simulink model "Evaluation"  (Simulink 7.6)
settings: Solver=ode45  StartTime=0.0  StopTime=10.0  RelTol=1e-3
libraries: powerlib_extras x1, simulink x1
settings Model: Creator=Zsolt  LastModifiedBy=Zsolt
settings HardwareCC: TargetIntDivRoundTo=Zero  TargetEndianess=LittleEndian  TargetHWDeviceType=MATLAB Host  ProdEqTarget=off
settings RTWCC: SystemTargetFile=rsim.tlc  TemplateMakefile=rsim_default_tmf  Description=Rapid Simulation Target  ProcessScript=rsim_make_rtw_hook
settings RSimTargetCC: TargetFunctionLibrary=ANSI_C  ERTMultiwordTypeDef=System defined  ERTCodeCoverageTool=None  ERTMultiwordLength=256  IsPILTarget=off  EnableShiftOperators=on  PortableWordSizes=off

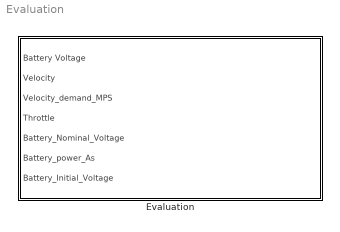
== system Evaluation ==
  Evaluation : Subsystem

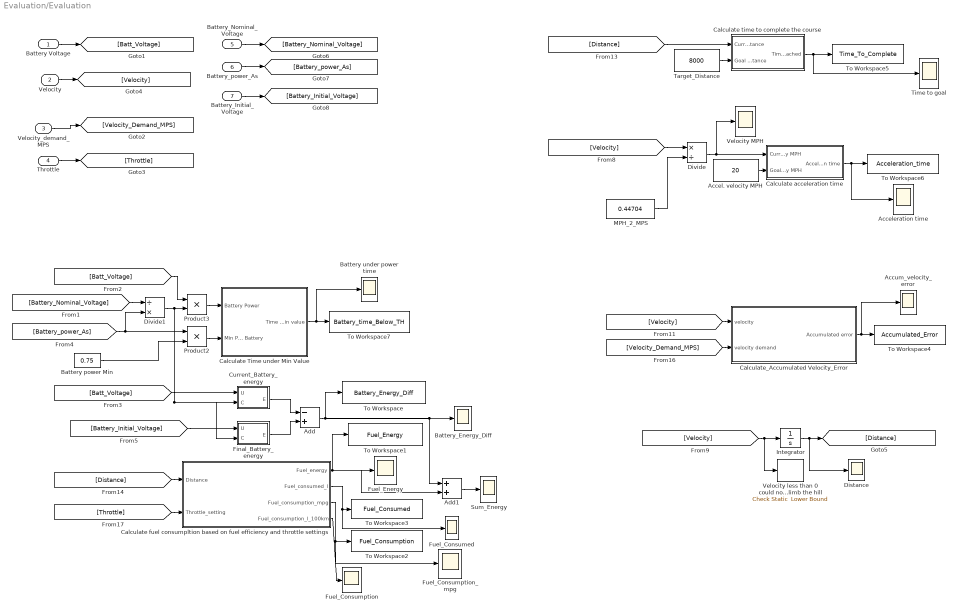
== system Evaluation/Evaluation ==
  Battery Voltage : Inport
  Velocity : Inport  Port=2
  Velocity_demand_MPS : Inport  Port=3
  Throttle : Inport  Port=4
  Battery_Nominal_Voltage : Inport  Port=5
  Battery_power_As : Inport  Port=6
  Battery_Initial_Voltage : Inport  Port=7
  Accel. velocity MPH : Constant  Value=20
  Acceleration time : Scope
      settings: TimeRange=500  YMin=0  YMax=10  SaveName=ScopeData15
  Accum_velocity_error : Scope
      settings: TimeRange=500  YMin=0  YMax=500  SaveName=ScopeData6
  Add : Sum  Inputs=-+
  Add1 : Sum
  Battery power Min : Constant  Value=0.75
  Battery under power time : Scope
      settings: TimeRange=500  YMin=0  YMax=400
  Battery_Energy_Diff : Scope
      settings: TimeRange=500  YMin=-500000  YMax=2000000  SaveName=ScopeData20
  Calculate Time under Min Value : Subsystem
  Calculate acceleration time : Subsystem
  Calculate time to complete the course : Subsystem
  Calculate fuel consumpltion based on fuel efficiency and throttle settings : Subsystem
  Calculate_Accumulated Velocity_Error : Subsystem
  Current_Battery_energy : Subsystem
  Distance : Scope
      settings: TimeRange=500  YMin=0  YMax=12000  SaveName=ScopeData8
  Divide : Product  Inputs=*/
  Divide1 : Product  Inputs=/*
  Final_Battery_energy : Subsystem
  Fuel_Consumed : Scope
      settings: TimeRange=500  YMin=0  YMax=20  SaveName=ScopeData21
  Fuel_Consumption : Scope
      settings: TimeRange=500  YMin=0  YMax=4000  SaveName=ScopeData22
  Fuel_Consumption_mpg : Scope
      settings: TimeRange=500  YMin=0  YMax=2  SaveName=ScopeData23
  Fuel_Energy : Scope
      settings: TimeRange=500  YMin=0  YMax=300000000  SaveName=ScopeData24
  Integrator : Integrator
  MPH_2_MPS : Constant  Value=0.44704
  Product2 : Product  RndMeth=Zero
  Product3 : Product  RndMeth=Zero
  Sum_Energy : Scope
      settings: TimeRange=500  YMin=0  YMax=14000  SaveName=ScopeData25
  Target_Distance : Constant  Value=8000
  Time to goal : Scope
      settings: TimeRange=500  YMin=0  YMax=500  SaveName=ScopeData5
  To Workspace : ToWorkspace  VariableName=Battery_Energy_Diff  SampleTime=-1  SaveFormat=Structure
  To Workspace1 : ToWorkspace  VariableName=Fuel_Energy  SampleTime=-1  SaveFormat=Structure
  To Workspace2 : ToWorkspace  VariableName=Fuel_Consumption  SampleTime=-1  SaveFormat=Structure
  To Workspace3 : ToWorkspace  VariableName=Fuel_Consumed  SampleTime=-1  SaveFormat=Structure
  To Workspace4 : ToWorkspace  VariableName=Accumulated_Error  SampleTime=-1  SaveFormat=Structure
  To Workspace5 : ToWorkspace  VariableName=Time_To_Complete  SampleTime=-1  SaveFormat=Structure
  To Workspace6 : ToWorkspace  VariableName=Acceleration_time  SampleTime=-1  SaveFormat=Structure
  To Workspace7 : ToWorkspace  VariableName=Battery_time_Below_TH  SampleTime=-1  SaveFormat=Structure
  Velocity MPH : Scope
      settings: TimeRange=500  YMin=0  YMax=60  SaveName=ScopeData13
  Velocity less than 0 could not climb the hill : simulink/Model Verification/Check Static  Lower Bound  Description=0 <= u  SystemSampleTime=-1  min=0  min_included=on  enabled=on  stopWhenAssertionFail=on  export=off  icon=graphic
  wires:
  MPH_2_MPS/1 -> Divide/2
  [Velocity] -> Divide/1
  Divide/1 -> Calculate acceleration time/1(Current Velocity MPH), Velocity MPH/1
  Calculate acceleration time/1(Acceleration time) -> Acceleration time/1, To Workspace6/1
  Accel. velocity MPH/1 -> Calculate acceleration time/2(Goal Velocity MPH)
  Product3/1 -> Calculate Time under Min Value/1(Battery Power)
  Battery power Min/1 -> Product2/2
  [Battery_power_As] -> Product2/1, Divide1/2
  Product2/1 -> Calculate Time under Min Value/2(Min Power in Battery)
  Calculate Time under Min Value/1(Time under Min value) -> Battery under power time/1, To Workspace7/1
  Calculate fuel consumpltion based on fuel efficiency and throttle settings/3(Fuel_consumption_mpg) -> Fuel_Consumption_mpg/1, To Workspace2/1
  Calculate fuel consumpltion based on fuel efficiency and throttle settings/2(Fuel_consumed_l) -> Fuel_Consumed/1, To Workspace3/1
  Calculate fuel consumpltion based on fuel efficiency and throttle settings/1(Fuel_energy) -> Fuel_Energy/1, To Workspace1/1, Add1/2
  Calculate fuel consumpltion based on fuel efficiency and throttle settings/4(Fuel_consumption_l_100km) -> Fuel_Consumption/1
  Add1/1 -> Sum_Energy/1
  Add/1 -> Battery_Energy_Diff/1, To Workspace/1, Add1/1
  Final_Battery_energy/1(E) -> Add/2
  Current_Battery_energy/1(E) -> Add/1
  [Battery_Initial_Voltage] -> Final_Battery_energy/1(U)
  [Batt_Voltage] -> Current_Battery_energy/1(U)
  [Distance] -> Calculate fuel consumpltion based on fuel efficiency and throttle settings/1(Distance)
  [Batt_Voltage] -> Product3/1
  Divide1/1 -> Product3/2, Final_Battery_energy/2(C), Current_Battery_energy/2(C)
  [Battery_Nominal_Voltage] -> Divide1/1
  [Throttle] -> Calculate fuel consumpltion based on fuel efficiency and throttle settings/2(Throttle_setting)
  Calculate time to complete the course/1(Time when reached) -> Time to goal/1, To Workspace5/1
  Target_Distance/1 -> Calculate time to complete the course/2(Goal Distance)
  [Distance] -> Calculate time to complete the course/1(Current Distance)
  Calculate_Accumulated Velocity_Error/1(Accumulated error) -> Accum_velocity_error/1, To Workspace4/1
  [Velocity] -> Calculate_Accumulated Velocity_Error/1(velocity)
  [Velocity_Demand_MPS] -> Calculate_Accumulated Velocity_Error/2(velocity demand)
  [Velocity] -> Integrator/1, Velocity less than 0 could not climb the hill/1
  Integrator/1 -> [Distance], Distance/1
  Battery Voltage/1 -> [Batt_Voltage]
  Velocity/1 -> [Velocity]
  Velocity_demand_MPS/1 -> [Velocity_Demand_MPS]
  Throttle/1 -> [Throttle]
  Battery_Nominal_Voltage/1 -> [Battery_Nominal_Voltage]
  Battery_power_As/1 -> [Battery_power_As]
  Battery_Initial_Voltage/1 -> [Battery_Initial_Voltage]

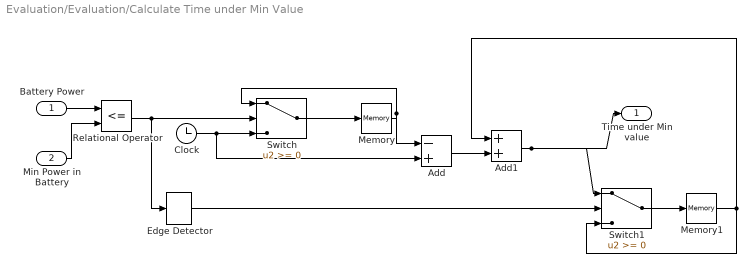
== system Evaluation/Evaluation/Calculate Time under Min Value ==
  Battery Power : Inport
  Min Power in Battery : Inport  Port=2
  Add : Sum  Inputs=-+
  Add1 : Sum
  Clock : Clock
      settings: Decimation=10
  Edge Detector : powerlib_extras/Control  Blocks/Edge Detector  DialogController=POWERSYS.PowerSysDialog  SystemSampleTime=-1  model=Falling  ic=0
  Memory : Memory
  Memory1 : Memory
  Relational Operator : RelationalOperator  Operator=<=  OutDataTypeStr=boolean
  Switch : Switch
  Switch1 : Switch
  Time under Min value : Outport
  wires:
  Switch/1 -> Memory/1
  Memory/1 -> Switch/1, Add/1
  Relational Operator/1 -> Switch/2, Edge Detector/1
  Clock/1 -> Switch/3, Add/2
  Add/1 -> Add1/2
  Switch1/1 -> Memory1/1
  Edge Detector/1 -> Switch1/2
  Memory1/1 -> Switch1/3, Add1/1
  Add1/1 -> Switch1/1, Time under Min value/1
  Battery Power/1 -> Relational Operator/1
  Min Power in Battery/1 -> Relational Operator/2

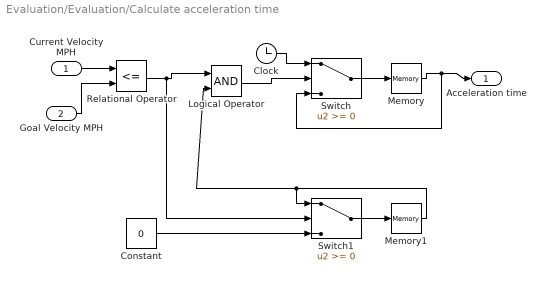
== system Evaluation/Evaluation/Calculate acceleration time ==
  Current Velocity MPH : Inport
  Goal Velocity MPH : Inport  Port=2
  Clock : Clock
      settings: Decimation=10
  Constant : Constant  Value=0
  Logical Operator : Logic  AllPortsSameDT=off  OutDataTypeStr=boolean
  Memory : Memory
  Memory1 : Memory  X0=1
  Relational Operator : RelationalOperator  Operator=<=  OutDataTypeStr=boolean
  Switch : Switch
  Switch1 : Switch
  Acceleration time : Outport
  wires:
  Goal Velocity MPH/1 -> Relational Operator/2
  Current Velocity MPH/1 -> Relational Operator/1
  Memory/1 -> Acceleration time/1, Switch/3
  Switch/1 -> Memory/1
  Memory1/1 -> Switch1/1, Logical Operator/2
  Switch1/1 -> Memory1/1
  Relational Operator/1 -> Logical Operator/1, Switch1/2
  Logical Operator/1 -> Switch/2
  Constant/1 -> Switch1/3
  Clock/1 -> Switch/1

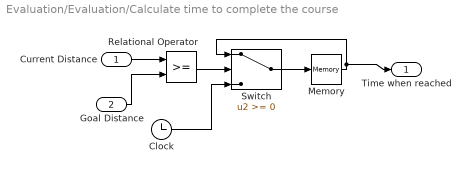
== system Evaluation/Evaluation/Calculate time to complete the course ==
  Current Distance : Inport
  Goal Distance : Inport  Port=2
  Clock : Clock
      settings: Decimation=10
  Memory : Memory
  Relational Operator : RelationalOperator  OutDataTypeStr=boolean
  Switch : Switch
  Time when reached : Outport
  wires:
  Switch/1 -> Memory/1
  Memory/1 -> Switch/1, Time when reached/1
  Relational Operator/1 -> Switch/2
  Clock/1 -> Switch/3
  Current Distance/1 -> Relational Operator/1
  Goal Distance/1 -> Relational Operator/2

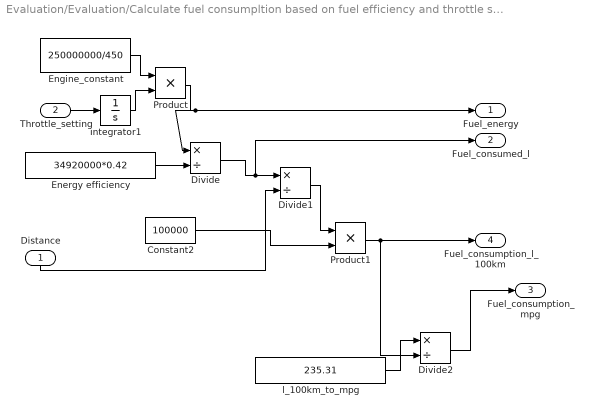
== system Evaluation/Evaluation/Calculate fuel consumpltion based on fuel efficiency and throttle settings ==
  Distance : Inport
  Throttle_setting : Inport  Port=2
  Constant2 : Constant  Value=100000
  Divide : Product  Inputs=*/
  Divide1 : Product  Inputs=*/
  Divide2 : Product  Inputs=*/
  Energy efficiency : Constant  Value=34920000*0.42
  Engine_constant : Constant  Value=250000000/450
  Integrator1 : Integrator
  Product : Product  RndMeth=Zero
  Product1 : Product  RndMeth=Zero
  l_100km_to_mpg : Constant  Value=235.31
  Fuel_energy : Outport
  Fuel_consumed_l : Outport  Port=2
  Fuel_consumption_mpg : Outport  Port=3
  Fuel_consumption_l_100km : Outport  Port=4
  wires:
  Integrator1/1 -> Product/2
  Product/1 -> Divide/1, Fuel_energy/1
  Engine_constant/1 -> Product/1
  Energy efficiency/1 -> Divide/2
  Divide/1 -> Divide1/1, Fuel_consumed_l/1
  Divide1/1 -> Product1/1
  Constant2/1 -> Product1/2
  Throttle_setting/1 -> Integrator1/1
  Distance/1 -> Divide1/2
  Product1/1 -> Fuel_consumption_l_100km/1, Divide2/2
  Divide2/1 -> Fuel_consumption_mpg/1
  l_100km_to_mpg/1 -> Divide2/1

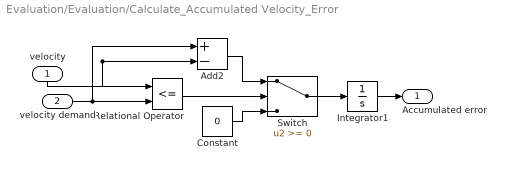
== system Evaluation/Evaluation/Calculate_Accumulated Velocity_Error ==
  velocity : Inport
  velocity demand : Inport  Port=2
  Add2 : Sum  Inputs=+-
  Constant : Constant  Value=0
  Integrator1 : Integrator
  Relational Operator : RelationalOperator  Operator=<=  OutDataTypeStr=boolean
  Switch : Switch
  Accumulated error : Outport
  wires:
  Relational Operator/1 -> Switch/2
  Constant/1 -> Switch/3
  Add2/1 -> Switch/1
  Switch/1 -> Integrator1/1
  velocity/1 -> Relational Operator/1, Add2/2
  velocity demand/1 -> Relational Operator/2, Add2/1
  Integrator1/1 -> Accumulated error/1

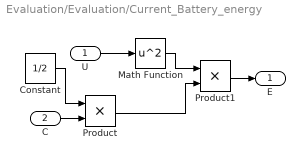
== system Evaluation/Evaluation/Current_Battery_energy ==
  U : Inport
  C : Inport  Port=2
  Constant : Constant  Value=1/2
  Math Function : Math  Operator=square  SaturateOnIntegerOverflow=on
  Product : Product  RndMeth=Zero
  Product1 : Product  RndMeth=Zero
  E : Outport
  wires:
  Constant/1 -> Product/1
  Product/1 -> Product1/2
  Math Function/1 -> Product1/1
  U/1 -> Math Function/1
  Product1/1 -> E/1
  C/1 -> Product/2

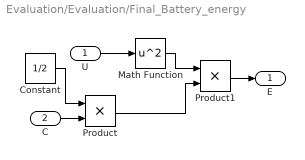
== system Evaluation/Evaluation/Final_Battery_energy ==
  U : Inport
  C : Inport  Port=2
  Constant : Constant  Value=1/2
  Math Function : Math  Operator=square  SaturateOnIntegerOverflow=on
  Product : Product  RndMeth=Zero
  Product1 : Product  RndMeth=Zero
  E : Outport
  wires:
  C/1 -> Product/2
  Product1/1 -> E/1
  U/1 -> Math Function/1
  Math Function/1 -> Product1/1
  Product/1 -> Product1/2
  Constant/1 -> Product/1
